simulink model "bote"  (R2024a)
settings: Solver=VariableStepAuto  StartTime=0.0  StopTime=10000.0  RelTol=1e-3
libraries: simulink x1
settings Model: Creator=klyx  LastModifiedBy=Eugen
settings RTWCC: GPUComputeCapability=3.5

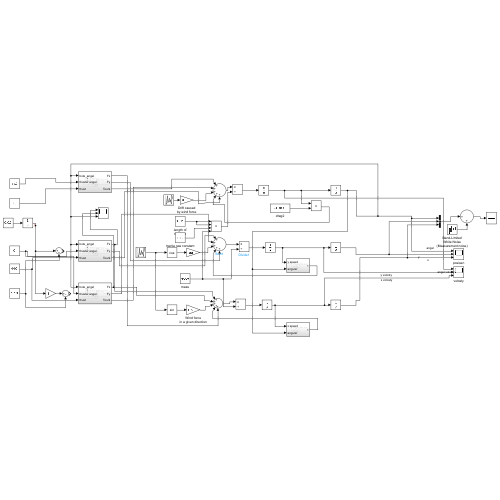
[thumbnail: Simulink's stored preview of the top-level diagram]
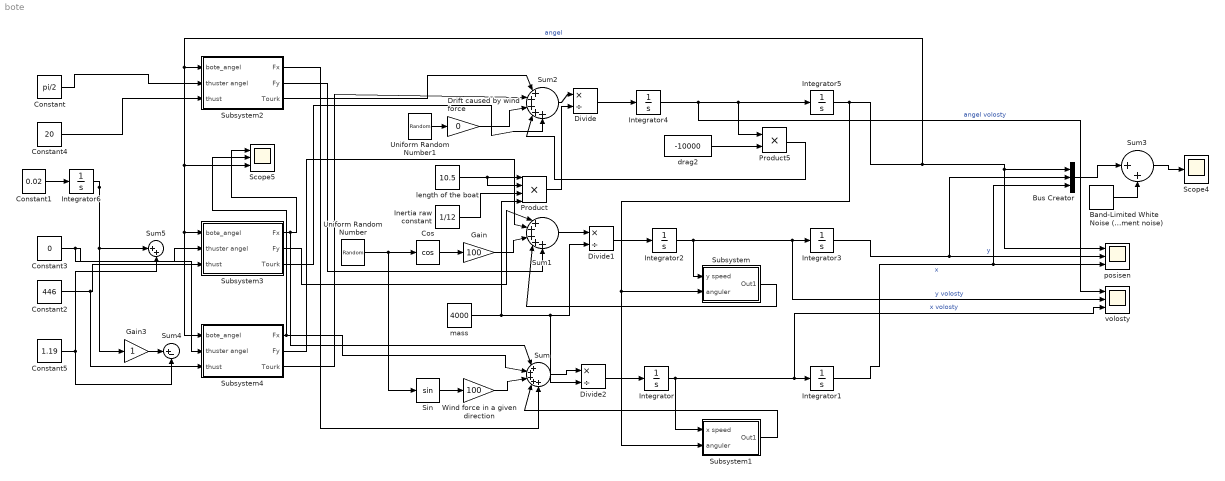
== system bote ==
  Band-Limited White Noise (Measurement noise) : simulink/Sources/Band-Limited White Noise  Cov=[0.01]  Ts=0.1  seed=[23341]
  Bus Creator : BusCreator  Inputs=3
  Constant : Constant  Value=pi/2
  Constant1 : Constant  Value=0.02
  Constant2 : Constant  Value=446
  Constant3 : Constant  Value=0
  Constant4 : Constant  Value=20
  Constant5 : Constant  Value=1.19
  Cos : Trigonometry  Operator=cos
  Divide : Product  Inputs=*/
  Divide1 : Product  Inputs=*/
  Divide2 : Product  Inputs=*/
  Drift caused by wind force : Gain  Gain=0
  Gain : Gain  Gain=100
  Gain3 : Gain
  Inertia raw constant : Constant  Value=1/12
  Integrator{,1..5} (6 alike) : Integrator
  Integrator6 : Integrator  InitialCondition=pi/2
  Product : Product  Inputs=4
  Product5 : Product
  Scope4 : Scope
  Scope5 : Scope  NumInputPorts=3
  Sin : Trigonometry
  Subsystem : Subsystem
  Subsystem1 : Subsystem
  Subsystem2 : Subsystem
  Subsystem3 : Subsystem
  Subsystem4 : Subsystem
  Sum : Sum  Inputs=|+++++
  Sum1 : Sum  Inputs=|+++++
  Sum2 : Sum  Inputs=|+++++
  Sum3 : Sum  Inputs=|++
  Sum4 : Sum  Inputs=|+-
  Sum5 : Sum  Inputs=|++
  Uniform Random Number : UniformRandomNumber  Minimum=0  Maximum=6.28  Seed=0.1  SampleTime=0.1
  Uniform Random Number1 : UniformRandomNumber  Minimum=0  Maximum=6.28  Seed=2  SampleTime=0.1
  Wind force in a given direction : Gain  Gain=100
  drag2 : Constant  Value=-10000
  length of the boat : Constant  Value=10.5
  mass : Constant  Value=4000
  posisen : Scope  NumInputPorts=3
  volosty : Scope  NumInputPorts=3
  wires:
  Integrator/1 -> Subsystem1/1(x speed), volosty/3, Integrator1/1  "x volosty"
  Divide2/1 -> Integrator/1
  Sin/1 -> Wind force in a given direction/1
  Integrator1/1 -> Bus Creator/3, posisen/3  "x"
  Cos/1 -> Gain/1
  mass/1 -> Product/4, Divide2/2, Divide1/2
  Sum1/1 -> Divide1/1
  Divide1/1 -> Integrator2/1
  Integrator3/1 -> Bus Creator/2, posisen/2  "y"
  Integrator2/1 -> Subsystem/1(y speed), volosty/2, Integrator3/1  "y volosty"
  Product5/1 -> Sum2/4
  length of the boat/1 -> Product/2, Product/1
  Sum2/1 -> Divide/1
  Integrator5/1 -> Subsystem1/2(anguler), Subsystem/2(anguler), Subsystem2/1(bote_angel), Subsystem4/1(bote_angel), Subsystem3/1(bote_angel), Scope5/3, posisen/1, Bus Creator/1  "angel"
  drag2/1 -> Product5/2
  Integrator4/1 -> volosty/1, Product5/1, Integrator5/1  "angel volosty"
  Divide/1 -> Integrator4/1
  Subsystem1/1(Out1) -> Sum/4
  Subsystem/1(Out1) -> Sum1/4
  Sum/1 -> Divide2/1
  Uniform Random Number/1 -> Sin/1, Cos/1
  Gain/1 -> Sum1/3
  Wind force in a given direction/1 -> Sum/3
  Bus Creator/1 -> Sum3/1
  Band-Limited White Noise (Measurement noise)/1 -> Sum3/2
  Sum3/1 -> Scope4/1
  Uniform Random Number1/1 -> Drift caused by wind force/1
  Product/1 -> Divide/2
  Inertia raw constant/1 -> Product/3
  Constant/1 -> Subsystem2/2(thuster angel)
  Subsystem2/3(Tourk) -> Sum2/1
  Subsystem3/3(Tourk) -> Sum2/5
  Subsystem4/3(Tourk) -> Sum2/2
  Subsystem4/1(Fx) -> Scope5/2, Sum/2
  Subsystem3/1(Fx) -> Sum/1, Scope5/1
  Subsystem4/2(Fy) -> Sum1/2
  Subsystem3/2(Fy) -> Sum1/1
  Constant1/1 -> Integrator6/1
  Drift caused by wind force/1 -> Sum2/3
  Constant4/1 -> Subsystem2/3(thust)
  Subsystem2/2(Fy) -> Sum1/5
  Subsystem2/1(Fx) -> Sum/5
  Constant2/1 -> Subsystem4/3(thust), Subsystem3/3(thust)
  Integrator6/1 -> Sum5/1, Gain3/1
  Gain3/1 -> Sum4/1
  Constant5/1 -> Sum5/2, Sum4/2
  Constant3/1 -> Subsystem4/2(thuster angel), Subsystem3/2(thuster angel)

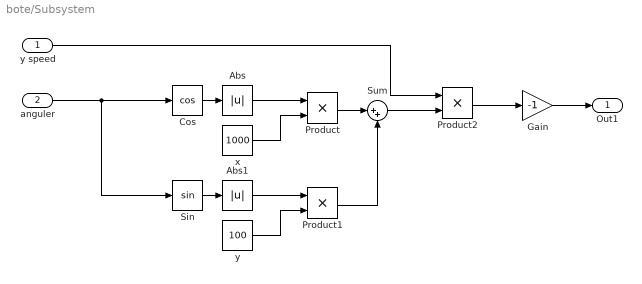
== system bote/Subsystem ==
  y speed : Inport
  anguler : Inport  Port=2
  Abs : Abs  SaturateOnIntegerOverflow=off
  Abs1 : Abs  SaturateOnIntegerOverflow=off
  Cos : Trigonometry  Operator=cos
  Gain : Gain  Gain=-1
  Product : Product
  Product1 : Product
  Product2 : Product
  Sin : Trigonometry
  Sum : Sum  Inputs=|++
  x : Constant  Value=1000
  y : Constant  Value=100
  Out1 : Outport
  wires:
  Product1/1 -> Sum/2
  Abs1/1 -> Product1/1
  Abs/1 -> Product/1
  Cos/1 -> Abs/1
  Product2/1 -> Gain/1
  Gain/1 -> Out1/1
  anguler/1 -> Sin/1, Cos/1
  Product/1 -> Sum/1
  x/1 -> Product/2
  y/1 -> Product1/2
  Sum/1 -> Product2/2
  Sin/1 -> Abs1/1
  y speed/1 -> Product2/1

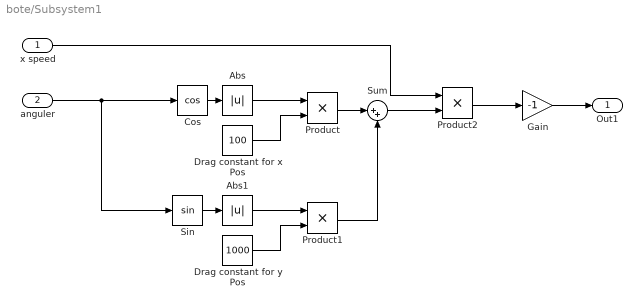
== system bote/Subsystem1 ==
  x speed : Inport
  anguler : Inport  Port=2
  Abs : Abs  SaturateOnIntegerOverflow=off
  Abs1 : Abs  SaturateOnIntegerOverflow=off
  Cos : Trigonometry  Operator=cos
  Drag constant for x Pos : Constant  Value=100
  Drag constant for y Pos : Constant  Value=1000
  Gain : Gain  Gain=-1
  Product : Product
  Product1 : Product
  Product2 : Product
  Sin : Trigonometry
  Sum : Sum  Inputs=|++
  Out1 : Outport
  wires:
  Product1/1 -> Sum/2
  Abs1/1 -> Product1/1
  Abs/1 -> Product/1
  Cos/1 -> Abs/1
  Product2/1 -> Gain/1
  Gain/1 -> Out1/1
  anguler/1 -> Sin/1, Cos/1
  Product/1 -> Sum/1
  Drag constant for x Pos/1 -> Product/2
  Drag constant for y Pos/1 -> Product1/2
  Sum/1 -> Product2/2
  Sin/1 -> Abs1/1
  x speed/1 -> Product2/1

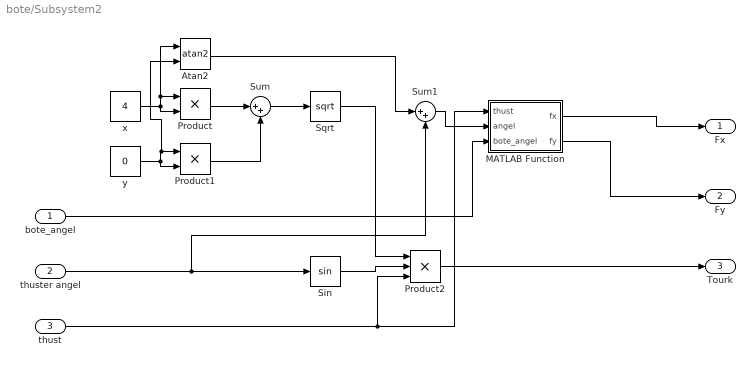
== system bote/Subsystem2 ==
  bote_angel : Inport
  thuster angel : Inport  Port=2
  thust : Inport  Port=3
  Atan2 : Trigonometry  Operator=atan2
  MATLAB Function : MATLAB Function  TreatAsAtomicUnit=on
  Product : Product
  Product1 : Product
  Product2 : Product  Inputs=3
  Sin : Trigonometry
  Sqrt : Sqrt
  Sum : Sum  Inputs=|++
  Sum1 : Sum  Inputs=|++
  x : Constant  Value=4
  y : Constant  Value=0
  Fx : Outport
  Fy : Outport  Port=2
  Tourk : Outport  Port=3
  wires:
  Sin/1 -> Product2/2
  Product1/1 -> Sum/2
  y/1 -> Product1/2, Atan2/2, Product1/1
  Product/1 -> Sum/1
  thuster angel/1 -> Sum1/2, Sin/1
  thust/1 -> MATLAB Function/1(thust), Product2/3
  bote_angel/1 -> MATLAB Function/3(bote_angel)
  MATLAB Function/1(fx) -> Fx/1
  MATLAB Function/2(fy) -> Fy/1
  Sum/1 -> Sqrt/1
  Product2/1 -> Tourk/1
  Sqrt/1 -> Product2/1
  x/1 -> Atan2/1, Product/1, Product/2
  Atan2/1 -> Sum1/1
  Sum1/1 -> MATLAB Function/2(angel)

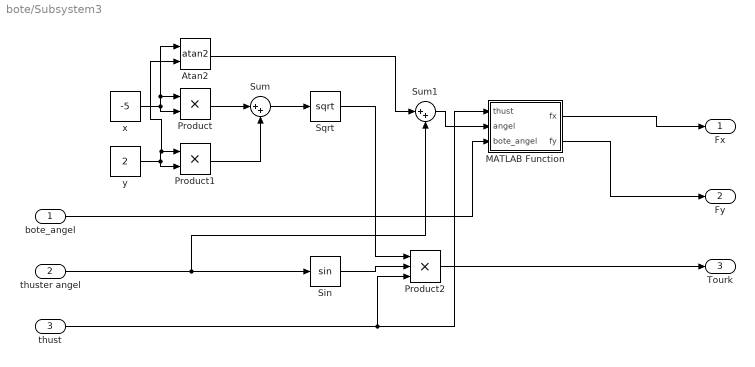
== system bote/Subsystem3 ==
  bote_angel : Inport
  thuster angel : Inport  Port=2
  thust : Inport  Port=3
  Atan2 : Trigonometry  Operator=atan2
  MATLAB Function : MATLAB Function  TreatAsAtomicUnit=on
  Product : Product
  Product1 : Product
  Product2 : Product  Inputs=3
  Sin : Trigonometry
  Sqrt : Sqrt
  Sum : Sum  Inputs=|++
  Sum1 : Sum  Inputs=|++
  x : Constant  Value=-5
  y : Constant  Value=2
  Fx : Outport
  Fy : Outport  Port=2
  Tourk : Outport  Port=3
  wires:
  Sin/1 -> Product2/2
  Product1/1 -> Sum/2
  y/1 -> Product1/2, Atan2/2, Product1/1
  Product/1 -> Sum/1
  thuster angel/1 -> Sum1/2, Sin/1
  thust/1 -> MATLAB Function/1(thust), Product2/3
  bote_angel/1 -> MATLAB Function/3(bote_angel)
  MATLAB Function/1(fx) -> Fx/1
  MATLAB Function/2(fy) -> Fy/1
  Sum/1 -> Sqrt/1
  Product2/1 -> Tourk/1
  Sqrt/1 -> Product2/1
  x/1 -> Atan2/1, Product/1, Product/2
  Atan2/1 -> Sum1/1
  Sum1/1 -> MATLAB Function/2(angel)

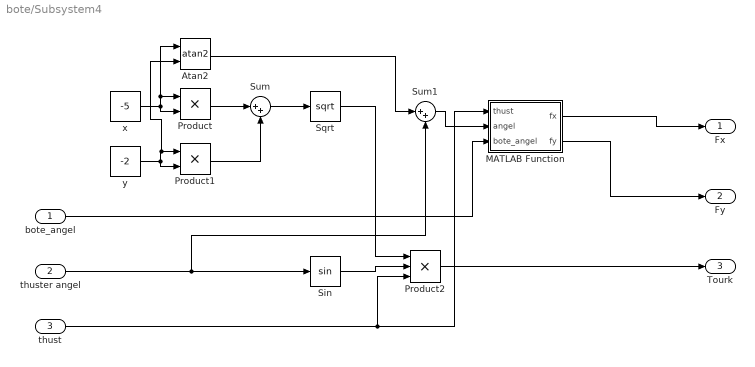
== system bote/Subsystem4 ==
  bote_angel : Inport
  thuster angel : Inport  Port=2
  thust : Inport  Port=3
  Atan2 : Trigonometry  Operator=atan2
  MATLAB Function : MATLAB Function  TreatAsAtomicUnit=on
  Product : Product
  Product1 : Product
  Product2 : Product  Inputs=3
  Sin : Trigonometry
  Sqrt : Sqrt
  Sum : Sum  Inputs=|++
  Sum1 : Sum  Inputs=|++
  x : Constant  Value=-5
  y : Constant  Value=-2
  Fx : Outport
  Fy : Outport  Port=2
  Tourk : Outport  Port=3
  wires:
  Sin/1 -> Product2/2
  Product1/1 -> Sum/2
  y/1 -> Product1/2, Atan2/2, Product1/1
  Product/1 -> Sum/1
  thuster angel/1 -> Sum1/2, Sin/1
  thust/1 -> MATLAB Function/1(thust), Product2/3
  bote_angel/1 -> MATLAB Function/3(bote_angel)
  MATLAB Function/1(fx) -> Fx/1
  MATLAB Function/2(fy) -> Fy/1
  Sum/1 -> Sqrt/1
  Product2/1 -> Tourk/1
  Sqrt/1 -> Product2/1
  x/1 -> Atan2/1, Product/1, Product/2
  Atan2/1 -> Sum1/1
  Sum1/1 -> MATLAB Function/2(angel)

== matlab function bote/Subsystem3/MATLAB Function ==
  data: thust input; fx output; angel input; bote_angel input; fy output
function [fx,fy] = fcn(thust, angel, bote_angel)

Rx = [cos(bote_angel) -sin(bote_angel); sin(bote_angel) cos(bote_angel)];
f = [sin(angel); cos(angel)];
mf = (Rx*f)*thust*(-1);
fx = mf(1);
fy = mf(2);

== matlab function bote/Subsystem2/MATLAB Function ==
  data: thust input; fx output; angel input; bote_angel input; fy output
function [fx,fy] = fcn(thust, angel, bote_angel)

Rx = [cos(bote_angel) -sin(bote_angel); sin(bote_angel) cos(bote_angel)];
f = [sin(angel); cos(angel)];
mf = (Rx*f)*thust;
fx = mf(1);
fy = mf(2);

== matlab function bote/Subsystem4/MATLAB Function ==
  data: thust input; fx output; angel input; bote_angel input; fy output
function [fx,fy] = fcn(thust, angel, bote_angel)

Rx = [cos(bote_angel) -sin(bote_angel); sin(bote_angel) cos(bote_angel)];
f = [sin(angel); cos(angel)];
mf = (Rx*f)*thust*(-1);
fx = mf(1);
fy = mf(2);
